simulink model "trab2_estabilidade"  (R2023a)
settings: Solver=VariableStepAuto  StartTime=0.0  StopTime=10.0  RelTol=1e-3
values from neighbouring files (symbols this model uses):
  A = [[-3.333 0 -1.3333];[2 -2 0];[0 4.7727 -0.04545]]    [Controlador_t3.m]    (also in lab2_controle2.m = [[0 1 0];[981.0001 0 -2.8814];[0 0 -100]]; trab3_controle2.m; trabalho1_controle2.m = [[0 1];[0 0]])
  b = [0; 0; 100]    [lab2_controle2.m]    (also in trabalho1_controle2.m = [0;-0.294])
  c = [0 0 1]    [Controlador_t3.m]    (also in lab2_controle2.m = [1 0 0]; trab3_controle2.m; trabalho1_controle2.m = [1,0])
settings Model: Creator=wesle  LastModifiedBy=wesle

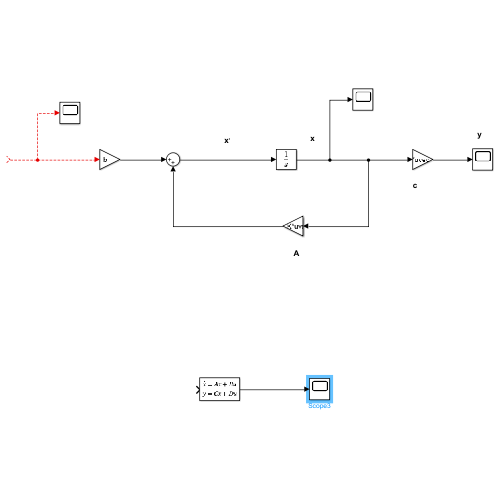
[thumbnail: Simulink's stored preview of the top-level diagram]
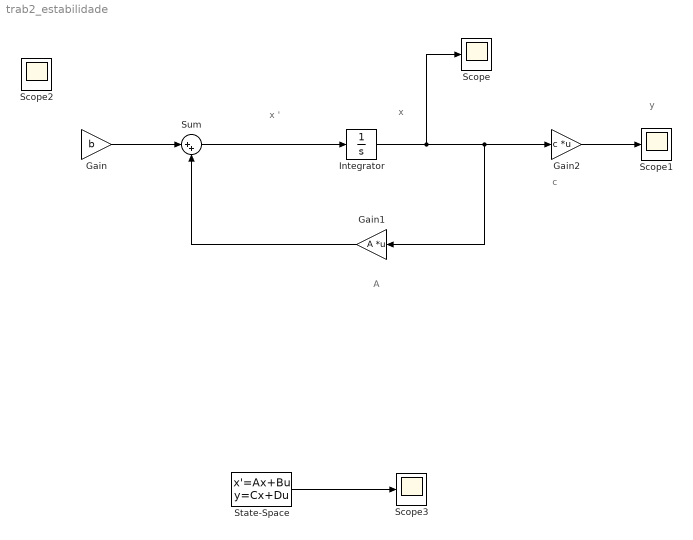
== system trab2_estabilidade ==
  note: c
  note: A
  note: x '
  note: x
  note: y
  Gain : Gain  Gain=b
  Gain1 : Gain  Gain=A  Multiplication=Matrix(K*u) (u vector)
  Gain2 : Gain  Gain=c  Multiplication=Matrix(K*u) (u vector)
  Integrator : Integrator  InitialCondition=[0.0005;0;0]
  Scope{,1..3} (4 alike) : Scope
  State-Space : StateSpace  A=A  B=b  C=c  D=0  InitialCondition=[0.0005;0;0]
  Sum : Sum  Inputs=|++
  wires:
  Sum/1 -> Integrator/1
  Gain/1 -> Sum/1
  Gain1/1 -> Sum/2
  ? -> Scope2/1, Gain/1
  Integrator/1 -> Scope/1, Gain1/1, Gain2/1
  Gain2/1 -> Scope1/1
  State-Space/1 -> Scope3/1
